simulink model "ee_EVchargerFaultAnalysis"  (R2024a)
settings: Solver=ode1be  StartTime=0.0  StopTime=.02  FixedStep=1e-7  MaxStep=1e-6  RelTol=1e-3  AbsTol=1e-3
PreLoadFcn:
  | systemLoadR=10;gridVoltage=415;gateDriveFault=zeros(6,1);
  | ee_EVchargerFaultAnalysis_ini
values from neighbouring files (symbols this model uses):
  gridFrequency = 50    [ee_EVchargerFaultAnalysis_ini.m]
undefined symbols (not defined in the file or in its folder): rectifier
libraries: fl_lib x13, nesl_utility_internal x12, ee_lib x10, eeTransforms x2, eePwmGeneratorTwoLevel x1, spsTHDLib x1, simulink_extras x1
(part 2 of 2)

== system ee_EVchargerFaultAnalysis/ControlUnit/ /Controller/q-axis current control ==
  e : Inport
  Integrator : Integrator  LimitOutput=on  UpperSaturationLimit=8  LowerSaturationLimit=-8
  Ki : Gain  Gain=1/rectifier.controller.CurrentT
  Kp : Gain  Gain=rectifier.controller.CurrentG
  Saturation : Saturate  UpperLimit=3  LowerLimit=-3
  Sum7 : Sum  Inputs=|++
  u : Outport  VectorParamsAs1DForOutWhenUnconnected=off
  wires:
  Ki/1 -> Integrator/1
  Kp/1 -> Sum7/1, Ki/1
  e/1 -> Kp/1
  Sum7/1 -> Saturation/1
  Saturation/1 -> u/1
  Integrator/1 -> Sum7/2

== matlab function ee_EVchargerFaultAnalysis/ControlUnit/PWM/MATLAB Function1 ==
  data: f input; actualFault_a output; actualFault_b output; actualFault_c output
function [actualFault_a,actualFault_b,actualFault_c] = faultInsert(f)
    actualFault_a=min(1,f(1,1)+f(2,1));
    actualFault_b=min(1,f(3,1)+f(4,1));
    actualFault_c=min(1,f(5,1)+f(6,1));
end

== matlab function ee_EVchargerFaultAnalysis/ControlUnit/PWM/MATLAB Function ==
  data: D output; duty input; num input
function D = fault(duty,num)
    % DutyCycle = [AH,AL,BH,BL,CH,CL]
    D=duty.*(1-num);
end
